simulink model "first_21_02_25"  (R2024b)
settings: Solver=VariableStepAuto  StartTime=0.0  StopTime=100  FixedStep=1e-3  MaxStep=1e-3  RelTol=0.1e-3
libraries: simulink x1
settings Model: Creator=claudio.rossi  LastModifiedBy=Franco
settings OptimizationCC: ReuseModelBlockBuffer=off
settings RTWCC: GPUComputeCapability=3.5

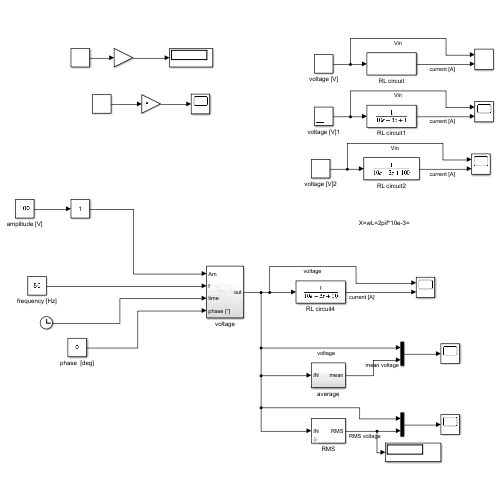
[thumbnail: Simulink's stored preview of the top-level diagram]
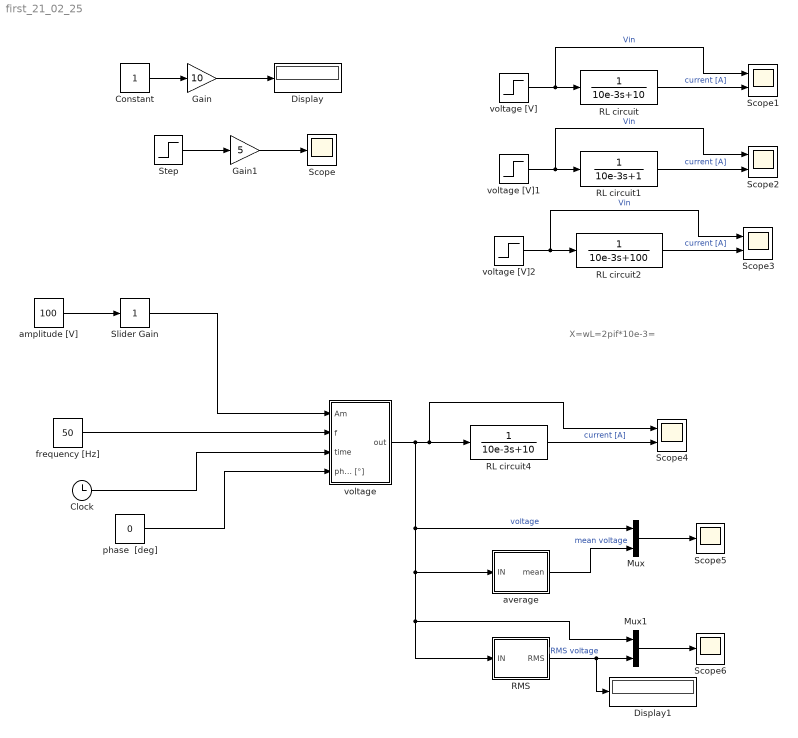
== system first_21_02_25 ==
  note: X=wL=2pif*10e-3=
  Clock : Clock
  Constant : Constant
  Display : Display
  Display1 : Display
  Gain : Gain  Gain=10
  Gain1 : Gain  Gain=5
  Mux : Mux  Inputs=2
  Mux1 : Mux  Inputs=2
  RL circuit : TransferFcn  Denominator=[10e-3 10]
  RL circuit1 : TransferFcn  Denominator=[10e-3 1]
  RL circuit2 : TransferFcn  Denominator=[10e-3 100]
  RL circuit4 : TransferFcn  Denominator=[10e-3 10]
  RMS : Subsystem  mask{period=20e-3}
      mask prompts: period "period [s]"
      mask DialogControl DescTextVar Prompt: calculates the RMS of a periodic function with period specified here
  Scope : Scope
  Scope{1..4} (4 alike) : Scope  NumInputPorts=2
  Scope5 : Scope
  Scope6 : Scope
  Slider Gain : simulink/Math Operations/Slider Gain  gain=1  low=0  high=2
  Step : Step  SampleTime=0
  amplitude [V] : Constant  Value=100
  average : Subsystem
  frequency [Hz] : Constant  Value=50
  phase  [deg] : Constant  Value=0
  voltage : Subsystem
  voltage [V] : Step  After=100  SampleTime=0
  voltage [V]1 : Step  After=100  SampleTime=0
  voltage [V]2 : Step  After=100  SampleTime=0
  wires:
  Constant/1 -> Gain/1
  Step/1 -> Gain1/1
  Gain/1 -> Display/1
  Gain1/1 -> Scope/1
  voltage [V]/1 -> Scope1/1, RL circuit/1  "Vin"
  RL circuit/1 -> Scope1/2  "current [A]"
  RL circuit1/1 -> Scope2/2  "current [A]"
  voltage [V]1/1 -> RL circuit1/1, Scope2/1  "Vin"
  voltage [V]2/1 -> Scope3/1, RL circuit2/1  "Vin"
  RL circuit2/1 -> Scope3/2  "current [A]"
  amplitude [V]/1 -> Slider Gain/1
  frequency [Hz]/1 -> voltage/2(f)
  Clock/1 -> voltage/3(time)
  phase  [deg]/1 -> voltage/4(phase [°])
  voltage/1(out) -> Mux/1, Mux1/1, RMS/1(IN), average/1(IN), Scope4/1, RL circuit4/1  "voltage"
  RL circuit4/1 -> Scope4/2  "current [A]"
  Slider Gain/1 -> voltage/1(Am)
  average/1(mean) -> Mux/2  "mean voltage"
  Mux/1 -> Scope5/1
  Mux1/1 -> Scope6/1
  RMS/1(RMS) -> Display1/1, Mux1/2  "RMS voltage"

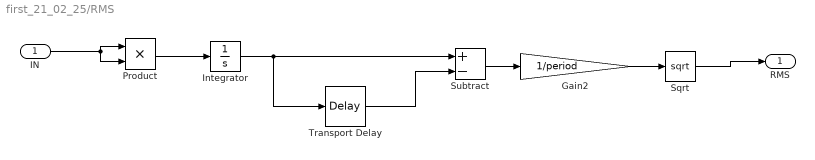
== system first_21_02_25/RMS ==
  IN : Inport
  Gain2 : Gain  Gain=1/period
  Integrator : Integrator
  Product : Product
  Sqrt : Sqrt
  Subtract : Sum  Inputs=+-
  Transport Delay : TransportDelay  DelayTime=period
  RMS : Outport
  wires:
  Transport Delay/1 -> Subtract/2
  Subtract/1 -> Gain2/1
  Integrator/1 -> Subtract/1, Transport Delay/1
  IN/1 -> Product/1, Product/2
  Product/1 -> Integrator/1
  Gain2/1 -> Sqrt/1
  Sqrt/1 -> RMS/1

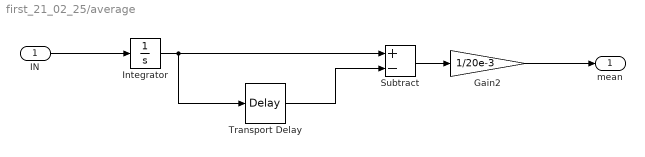
== system first_21_02_25/average ==
  IN : Inport
  Gain2 : Gain  Gain=1/20e-3
  Integrator : Integrator
  Subtract : Sum  Inputs=+-
  Transport Delay : TransportDelay  DelayTime=20e-3
  mean : Outport
  wires:
  Integrator/1 -> Transport Delay/1, Subtract/1
  Gain2/1 -> mean/1
  Subtract/1 -> Gain2/1
  Transport Delay/1 -> Subtract/2
  IN/1 -> Integrator/1

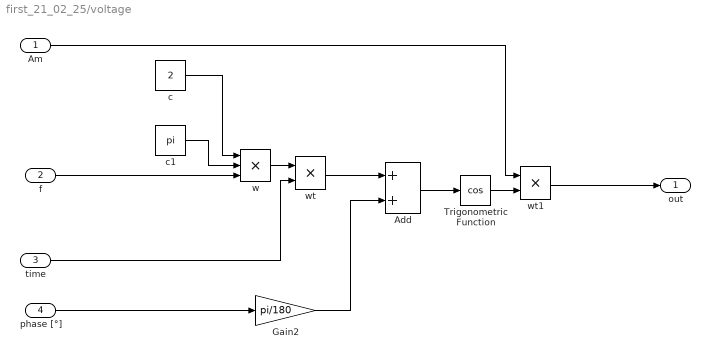
== system first_21_02_25/voltage ==
  Am : Inport
  f : Inport  Port=2
  time : Inport  Port=3
  phase [°] : Inport  Port=4
  Add : Sum
  Gain2 : Gain  Gain=pi/180
  Trigonometric Function : Trigonometry  Operator=cos
  c : Constant  Value=2
  c1 : Constant  Value=pi
  w : Product  Inputs=3
  wt : Product
  wt1 : Product
  out : Outport
  wires:
  wt/1 -> Add/1
  Add/1 -> Trigonometric Function/1
  phase [°]/1 -> Gain2/1
  c/1 -> w/1
  w/1 -> wt/1
  Trigonometric Function/1 -> wt1/2
  c1/1 -> w/2
  Gain2/1 -> Add/2
  wt1/1 -> out/1
  f/1 -> w/3
  time/1 -> wt/2
  Am/1 -> wt1/1
